simulink model "dspace"  (R2021b)
settings: Solver=FixedStepDiscrete  StartTime=0.0  StopTime=Inf  FixedStep=1e-3  RelTol=1e-3
PostLoadFcn:
  | , if any(exist('dsrtsu_mdlpostloadfcn', 'file') ~= 0), dsrtsu_mdlpostloadfcn('Execute', bdroot); end,
undefined symbols (not defined in the file): ami, amk1_setpoints_1, amk2_setpoints_1, amk3_setpoints_1, amk4_setpoints_1, as, digital, ebs, indicator, mcu_set_dbu_indicator_points, mcu_set_ecu_indicator_points, res_ntm_node_control
libraries: rtican x63, rti1401lib_dio_type3 x4, simulink x4, simulink_extras x1
(part 7 of 16)

== system dspace/CAN RX/amk4_actual_values_1 ==
  amk4_actual_values_11 : rtican/RTICAN Receive (RX)   Reserved1=[]  Reserved2=[]  Reserved3=[]  Reserved4=[]  SfcnMessage=[]  Msg_Struct=[]  BoardTypeNo=[]  BoardNo=[]  ChannelNo=[]  Parameters=[]  DialogFcn=[]  UnitName=[]  Revision=[]  UnitValues=[]  DSProperties=struct('RTI',struct('Version',uint32(5),'BlockType',struct('isSLSource',uint8(1),'isSLSink',uint8(1),'isHWSource',uint8(0),'isHWSink',uint8(0),'isSetup',uint8(0),'isInline',uint8(1),'isNonInline',uint8(0),'isInterrupt',uint8(0),'isChannelwise',uint8(0)),'IOBoardType','RTICAN','UnitType','MESSAGE','Identifier','RX','DialogType','MSVC','BlockSet','RTICAN','SlaveProcessor','CAN'))  RTIBlockInterface=struct('OutputPortsWidth',int32([1 1 1 1 1 1 1 1 1 1 1 1 1 1]),'OutputPortsActive',ones(1,14),'OutputPortsName',{{'amk4_system_ready','amk4_error','amk4_warning','amk4_status_quit_dc_on','amk4_status_dc_on','amk4_status_quit_inverter_on','amk4_status_inverter_on','amk4_status_derating','amk4_actual_velocity','amk4_torque_current','amk4_magnetizing_current',['RX status'],['RX time'],['RX delta time']}},'OutputPortsDataType',{{'SS_DOUBLE','SS_DOUBLE','SS_DOUBLE','SS_DOUBLE','SS_DOUBLE','SS_DOUBLE','SS_DOUBLE','SS_DOUBLE','SS_DOUBLE','SS_DOUBLE','SS_DOUBLE','SS_DOUBLE','SS_DOUBLE','SS_DOUBLE'}},'OutputPortsLabel',{{'amk4_system_ready','amk4_error','amk4_warning','amk4_status_quit_dc_on','amk4_status_dc_on','amk4_status_quit_inverter_on','amk4_status_inverter_on','amk4_status_derating','amk4_actual_velocity','amk4_torque_current','amk4_magnetizing_current','','',''}},'OutputPortsLabelMode','ON','InputPortsWidth',int32(0),'InputPortsActive',0,'DialogFcn','rtican_message_interface_gui','BlockDisplay',{{'','center'}},'IconTransparency','on','ParameterTunableNames',{{}},'InitLevel',3,'BlockName',struct('Token',{{'amk4_actual_values_1'}}),'SampleTime',{{-1}},'TriggerPort',{{'none'}},'EnablePort',{{'none'}})  RTIBlockParameters=struct('BoardTypeNo',{{1,'OFF',[]}},'BoardNo',{{1,'ON',[1 16]}},'ChannelNo',{{1,'ON',[1 2]}},'Parameters',{{struct('DataFileSupport',struct('DataFileSelectedMaster',1,'DataFileSelectedLocal',1,'DataFileName','c:\users\oscar\documents\github\sw_infrastructure\kthfspe_python\databases\can2.dbc|','DataFileDate',{{{['10-Jul-2022 04:24:51']}}},'SelectedFile','c:\users\oscar\documents\github\sw_infrastructure\kthfspe_python\databases\can2.dbc'),'Options',struct('StatusSelected',1,'TimeSelected',1,'DeltaTimeSelected',1,'BytePortSelected',0,'MessageLengthSelected',0,'TriggerPort',struct('Selected',0,'TriggerType',0),'UserCoding',struct('Selected',0,'InterfaceFile','UserDecodingFile','FcnName','UserDecodeFcn','InportSelected',0,'InportWidth',1,'OutportSelected',0,'OutportWidth',1),'EnablePortSelected',0,'SignalOnPortnameSelected',1,'UseRXService',0),'Message',struct('MsgOnBlocknameSelected',1,'MsgName','amk4_actual_values_1','MsgIdFormat',0,'MsgId',648,'MsgLength',8,'NumSignals',11,'SampleTime',-1,'Signal',struct('SgnName',{'amk4_system_ready','amk4_error','amk4_warning','amk4_status_quit_dc_on','amk4_status_dc_on','amk4_status_quit_inverter_on','amk4_status_inverter_on','amk4_status_derating','amk4_actual_velocity','amk4_torque_current','amk4_magnetizing_current'},'SgnStartBit',{8,9,10,11,12,13,14,15,16,32,48},'SgnLength',{1,1,1,1,1,1,1,1,16,16,16},'SgnType',{0,0,0,0,0,0,0,0,0,0,0},'ModeValue',{-1,-1,-1,-1,-1,-1,-1,-1,-1,-1,-1},'DataType',{0,0,0,0,0,0,0,0,1,1,1},'ByteLayout',{0,0,0,0,0,0,0,0,0,0,0},'Factor',{1,1,1,1,1,1,1,1,1,1,1},'Offset',{0,0,0,0,0,0,0,0,0,0,0},'SgnComment',{{''},{''},{''},{''},{''},{''},{''},{''},{''},{''},{''}},'SgnUnit',{'','','','','','','','','rpm','',''},'Min',{0,0,0,0,0,0,0,0,0,0,0},'Max',{0,0,0,0,0,0,0,0,0,0,0},'SLDataType',{'SS_DOUBLE','SS_DOUBLE','SS_DOUBLE','SS_DOUBLE','SS_DOUBLE','SS_DOUBLE','SS_DOUBLE','SS_DOUBLE','SS_DOUBLE','SS_DOUBLE','SS_DOUBLE'}),'MsgIdNumFormat',0,'MsgComment',{{['Periodic 5ms.']}}),'Version',1.2,'general',struct('isFromLib',0)),'OFF',[]}},'GroupId',{{struct('Group',{{'RTICAN'}},'No',2,'Behavior',{{'NAMECHANGE'}},'BlockType',{{'SINK'}},'NameChangeFlag',0),'OFF',[]}},'SFcnRTICANMessage',{{struct('MsgType','RX','SFcnPortType','Scalar','MsgName','amk4_actual_values_1','MsgIdFormat','STD','MsgId',648,'MsgLength',8,'NumSignals',11,'SampleTime',-1,'Signal',struct('SgnName',{'amk4_system_ready','amk4_error','amk4_warning','amk4_status_quit_dc_on','amk4_status_dc_on','amk4_status_quit_inverter_on','amk4_status_inverter_on','amk4_status_derating','amk4_actual_velocity','amk4_torque_current','amk4_magnetizing_current'},'SgnStartBit',{8,9,10,11,12,13,14,15,16,32,48},'SgnLength',{1,1,1,1,1,1,1,1,16,16,16},'SgnType',{'standard','standard','standard','standard','standard','standard','standard','standard','standard','standard','standard'},'ModeValue',{-1,-1,-1,-1,-1,-1,-1,-1,-1,-1,-1},'DataType',{['unsigned int'],['unsigned int'],['unsigned int'],['unsigned int'],['unsigned int'],['unsigned int'],['unsigned int'],['unsigned int'],['signed int'],['signed int'],['signed int']},'ByteLayout',{['little endian'],['little endian'],['little endian'],['little endian'],['little endian'],['little endian'],['little endian'],['little endian'],['little endian'],['little endian'],['little endian']},'Factor',{1,1,1,1,1,1,1,1,1,1,1},'Offset',{0,0,0,0,0,0,0,0,0,0,0},'SLDataType',{'SS_DOUBLE','SS_DOUBLE','SS_DOUBLE','SS_DOUBLE','SS_DOUBLE','SS_DOUBLE','SS_DOUBLE','SS_DOUBLE','SS_DOUBLE','SS_DOUBLE','SS_DOUBLE'}),'StatusSelected','yes','TimeSelected','yes','DeltaTimeSelected','yes','BytePortSelected','no','MessageLengthSelected','no','TriggerPort',struct('Selected','no','TriggerType',0),'UserCoding',struct('Selected','no','InterfaceFile','UserDecodingFile','FcnName','UserDecodeFcn','InportSelected','no','InportWidth',1,'OutportSelected','no','OutportWidth',1),'EnablePortSelected','no','UseRXService','no','BoardType','DS1','BoardNo',1,'ControllerNo',2),'OFF',[]}},'TLCFileName',{{'rtican_rx_message','OFF',[]}})  RTISFcnParameters=struct('SFcnRTICANMessage','struct','TLCFileName','char')  RTIBlockParaDefault=struct('BoardTypeNo',4302,'BoardNo',1,'ChannelNo',1,'Parameters',struct('DataFileSupport',struct('DataFileSelectedMaster',0,'DataFileSelectedLocal',0,'DataFileName','','DataFileDate','','SelectedFile',['<no file selected>']),'Options',struct('StatusSelected',1,'TimeSelected',1,'DeltaTimeSelected',1,'BytePortSelected',0,'MessageLengthSelected',0,'TriggerPort',struct('Selected',0,'TriggerType','rising'),'UserCoding',struct('Selected',0,'InterfaceFile','UserDecodingFile','FcnName','UserDecodeFcn','InportSelected',0,'InportWidth',1,'OutportSelected',0,'OutportWidth',1),'EnablePortSelected',0,'SignalOnPortnameSelected',1,'UseRXService',0),'Message',struct('MsgOnBlocknameSelected',0,'MsgName',['RX Message'],'MsgIdFormat',0,'MsgId',100,'MsgLength',8,'NumSignals',1,'SampleTime',-1,'Signal',struct('SgnName',['RX signal'],'SgnStartBit',0,'SgnLength',8,'SgnType',0,'ModeValue',-1,'DataType',0,'SLDataType','SS_DOUBLE','ByteLayout',0,'Factor',1,'Offset',0,'Min',0,'Max',255,'SgnComment',{{}},'SgnUnit',''),'MsgIdNumFormat',0,'MsgComment',{{''}}),'Version',1.2,'general',struct('isFromLib',1)),'GroupId',struct('Group',{{'RTICAN'}},'No',1,'Behavior',{{'NAMECHANGE'}},'BlockType',{{'SINK'}},'NameChangeFlag',0),'SFcnRTICANMessage',struct('MsgType','RX','MsgName',['RX Message'],'MsgIdFormat','STD','MsgId',100,'MsgLength',8,'NumSignals',1,'SampleTime',-1,'Signal',struct('SgnName',['RX signal'],'SgnStartBit',0,'SgnLength',8,'SgnType','standard','ModeValue',-1,'DataType',['unsigned int'],'ByteLayout',['little endian'],'SLDataType','SS_DOUBLE','Factor',1,'Offset',0),'StatusSelected','yes','TimeSelected','yes','DeltaTimeSelected','yes','BytePortSelected','no','MessageLengthSelected','no','EnablePortSelected','no','UserCoding',struct('Selected','no','InterfaceFile','UserDecodingFile','FcnName','UserDecodeFcn','InportSelected','no','InportWidth',1,'OutportSelected','no','OutportWidth',1),'TriggerPort',struct('Selected','no','TriggerType','rising'),'UseRXService','no','BoardType','DS4302','BoardNo',1,'ControllerNo',1,'SFcnPortType','Scalar'),'TLCFileName','rtican_rx_message')
      settings: AttributesFormatString=Group Id: RTICAN2\n  SourceProductName=dSPACE RTI CAN Blockset
  clock_time : Clock
  sub_time : Sum  Inputs=+-
  amk4_system_ready_bus : Outport  PortName=signals  Element=amk4_system_ready
  amk4_error_bus : Outport  PortName=signals  Element=amk4_error
  amk4_warning_bus : Outport  PortName=signals  Element=amk4_warning
  amk4_status_quit_dc_on_bus : Outport  PortName=signals  Element=amk4_status_quit_dc_on
  amk4_status_dc_on_bus : Outport  PortName=signals  Element=amk4_status_dc_on
  amk4_status_quit_inverter_on_bus : Outport  PortName=signals  Element=amk4_status_quit_inverter_on
  amk4_status_inverter_on_bus : Outport  PortName=signals  Element=amk4_status_inverter_on
  amk4_status_derating_bus : Outport  PortName=signals  Element=amk4_status_derating
  amk4_actual_velocity_bus : Outport  PortName=signals  Element=amk4_actual_velocity
  amk4_torque_current_bus : Outport  PortName=signals  Element=amk4_torque_current
  amk4_magnetizing_current_bus : Outport  PortName=signals  Element=amk4_magnetizing_current
  status : Outport  Port=2
  time : Outport  Port=3
  delta : Outport  Port=4
  wires:
  clock_time/1 -> sub_time/1
  sub_time/1 -> time/1
  amk4_actual_values_11/12 -> status/1
  amk4_actual_values_11/13 -> sub_time/2
  amk4_actual_values_11/14 -> delta/1
  amk4_actual_values_11/1 -> amk4_system_ready_bus/1  "amk4_system_ready"
  amk4_actual_values_11/2 -> amk4_error_bus/1  "amk4_error"
  amk4_actual_values_11/3 -> amk4_warning_bus/1  "amk4_warning"
  amk4_actual_values_11/4 -> amk4_status_quit_dc_on_bus/1  "amk4_status_quit_dc_on"
  amk4_actual_values_11/5 -> amk4_status_dc_on_bus/1  "amk4_status_dc_on"
  amk4_actual_values_11/6 -> amk4_status_quit_inverter_on_bus/1  "amk4_status_quit_inverter_on"
  amk4_actual_values_11/7 -> amk4_status_inverter_on_bus/1  "amk4_status_inverter_on"
  amk4_actual_values_11/8 -> amk4_status_derating_bus/1  "amk4_status_derating"
  amk4_actual_values_11/9 -> amk4_actual_velocity_bus/1  "amk4_actual_velocity"
  amk4_actual_values_11/10 -> amk4_torque_current_bus/1  "amk4_torque_current"
  amk4_actual_values_11/11 -> amk4_magnetizing_current_bus/1  "amk4_magnetizing_current"

== system dspace/CAN RX/amk4_actual_values_2 ==
  amk4_actual_values_21 : rtican/RTICAN Receive (RX)   Reserved1=[]  Reserved2=[]  Reserved3=[]  Reserved4=[]  SfcnMessage=[]  Msg_Struct=[]  BoardTypeNo=[]  BoardNo=[]  ChannelNo=[]  Parameters=[]  DialogFcn=[]  UnitName=[]  Revision=[]  UnitValues=[]  DSProperties=struct('RTI',struct('Version',uint32(5),'BlockType',struct('isSLSource',uint8(1),'isSLSink',uint8(1),'isHWSource',uint8(0),'isHWSink',uint8(0),'isSetup',uint8(0),'isInline',uint8(1),'isNonInline',uint8(0),'isInterrupt',uint8(0),'isChannelwise',uint8(0)),'IOBoardType','RTICAN','UnitType','MESSAGE','Identifier','RX','DialogType','MSVC','BlockSet','RTICAN','SlaveProcessor','CAN'))  RTIBlockInterface=struct('OutputPortsWidth',int32([1 1 1 1 1 1 1]),'OutputPortsActive',[1 1 1 1 1 1 1],'OutputPortsName',{{'amk4_temp_motor','amk4_temp_inverter','amk4_error_info','amk4_temp_igbt',['RX status'],['RX time'],['RX delta time']}},'OutputPortsDataType',{{'SS_DOUBLE','SS_DOUBLE','SS_DOUBLE','SS_DOUBLE','SS_DOUBLE','SS_DOUBLE','SS_DOUBLE'}},'OutputPortsLabel',{{'amk4_temp_motor','amk4_temp_inverter','amk4_error_info','amk4_temp_igbt','','',''}},'OutputPortsLabelMode','ON','InputPortsWidth',int32(0),'InputPortsActive',0,'DialogFcn','rtican_message_interface_gui','BlockDisplay',{{'','center'}},'IconTransparency','on','ParameterTunableNames',{{}},'InitLevel',3,'BlockName',struct('Token',{{'amk4_actual_values_2'}}),'SampleTime',{{-1}},'TriggerPort',{{'none'}},'EnablePort',{{'none'}})  RTIBlockParameters=struct('BoardTypeNo',{{1,'OFF',[]}},'BoardNo',{{1,'ON',[1 16]}},'ChannelNo',{{1,'ON',[1 2]}},'Parameters',{{struct('DataFileSupport',struct('DataFileSelectedMaster',1,'DataFileSelectedLocal',1,'DataFileName','c:\users\oscar\documents\github\sw_infrastructure\kthfspe_python\databases\can2.dbc|','DataFileDate',{{{['10-Jul-2022 04:24:51']}}},'SelectedFile','c:\users\oscar\documents\github\sw_infrastructure\kthfspe_python\databases\can2.dbc'),'Options',struct('StatusSelected',1,'TimeSelected',1,'DeltaTimeSelected',1,'BytePortSelected',0,'MessageLengthSelected',0,'TriggerPort',struct('Selected',0,'TriggerType',0),'UserCoding',struct('Selected',0,'InterfaceFile','UserDecodingFile','FcnName','UserDecodeFcn','InportSelected',0,'InportWidth',1,'OutportSelected',0,'OutportWidth',1),'EnablePortSelected',0,'SignalOnPortnameSelected',1,'UseRXService',0),'Message',struct('MsgOnBlocknameSelected',1,'MsgName','amk4_actual_values_2','MsgIdFormat',0,'MsgId',656,'MsgLength',8,'NumSignals',4,'SampleTime',-1,'Signal',struct('SgnName',{'amk4_temp_motor','amk4_temp_inverter','amk4_error_info','amk4_temp_igbt'},'SgnStartBit',{0,16,32,48},'SgnLength',{16,16,16,16},'SgnType',{0,0,0,0},'ModeValue',{-1,-1,-1,-1},'DataType',{1,1,0,1},'ByteLayout',{0,0,0,0},'Factor',{0.1,0.1,1,0.1},'Offset',{0,0,0,0},'SgnComment',{{''},{''},{''},{''}},'SgnUnit',{'C','C','','C'},'Min',{0,0,0,0},'Max',{0,0,0,0},'SLDataType',{'SS_DOUBLE','SS_DOUBLE','SS_DOUBLE','SS_DOUBLE'}),'MsgIdNumFormat',0,'MsgComment',{{['Periodic 5ms.']}}),'Version',1.2,'general',struct('isFromLib',0)),'OFF',[]}},'GroupId',{{struct('Group',{{'RTICAN'}},'No',2,'Behavior',{{'NAMECHANGE'}},'BlockType',{{'SINK'}},'NameChangeFlag',0),'OFF',[]}},'SFcnRTICANMessage',{{struct('MsgType','RX','SFcnPortType','Scalar','MsgName','amk4_actual_values_2','MsgIdFormat','STD','MsgId',656,'MsgLength',8,'NumSignals',4,'SampleTime',-1,'Signal',struct('SgnName',{'amk4_temp_motor','amk4_temp_inverter','amk4_error_info','amk4_temp_igbt'},'SgnStartBit',{0,16,32,48},'SgnLength',{16,16,16,16},'SgnType',{'standard','standard','standard','standard'},'ModeValue',{-1,-1,-1,-1},'DataType',{['signed int'],['signed int'],['unsigned int'],['signed int']},'ByteLayout',{['little endian'],['little endian'],['little endian'],['little endian']},'Factor',{0.1,0.1,1,0.1},'Offset',{0,0,0,0},'SLDataType',{'SS_DOUBLE','SS_DOUBLE','SS_DOUBLE','SS_DOUBLE'}),'StatusSelected','yes','TimeSelected','yes','DeltaTimeSelected','yes','BytePortSelected','no','MessageLengthSelected','no','TriggerPort',struct('Selected','no','TriggerType',0),'UserCoding',struct('Selected','no','InterfaceFile','UserDecodingFile','FcnName','UserDecodeFcn','InportSelected','no','InportWidth',1,'OutportSelected','no','OutportWidth',1),'EnablePortSelected','no','UseRXService','no','BoardType','DS1','BoardNo',1,'ControllerNo',2),'OFF',[]}},'TLCFileName',{{'rtican_rx_message','OFF',[]}})  RTISFcnParameters=struct('SFcnRTICANMessage','struct','TLCFileName','char')  RTIBlockParaDefault=struct('BoardTypeNo',4302,'BoardNo',1,'ChannelNo',1,'Parameters',struct('DataFileSupport',struct('DataFileSelectedMaster',0,'DataFileSelectedLocal',0,'DataFileName','','DataFileDate','','SelectedFile',['<no file selected>']),'Options',struct('StatusSelected',1,'TimeSelected',1,'DeltaTimeSelected',1,'BytePortSelected',0,'MessageLengthSelected',0,'TriggerPort',struct('Selected',0,'TriggerType','rising'),'UserCoding',struct('Selected',0,'InterfaceFile','UserDecodingFile','FcnName','UserDecodeFcn','InportSelected',0,'InportWidth',1,'OutportSelected',0,'OutportWidth',1),'EnablePortSelected',0,'SignalOnPortnameSelected',1,'UseRXService',0),'Message',struct('MsgOnBlocknameSelected',0,'MsgName',['RX Message'],'MsgIdFormat',0,'MsgId',100,'MsgLength',8,'NumSignals',1,'SampleTime',-1,'Signal',struct('SgnName',['RX signal'],'SgnStartBit',0,'SgnLength',8,'SgnType',0,'ModeValue',-1,'DataType',0,'SLDataType','SS_DOUBLE','ByteLayout',0,'Factor',1,'Offset',0,'Min',0,'Max',255,'SgnComment',{{}},'SgnUnit',''),'MsgIdNumFormat',0,'MsgComment',{{''}}),'Version',1.2,'general',struct('isFromLib',1)),'GroupId',struct('Group',{{'RTICAN'}},'No',1,'Behavior',{{'NAMECHANGE'}},'BlockType',{{'SINK'}},'NameChangeFlag',0),'SFcnRTICANMessage',struct('MsgType','RX','MsgName',['RX Message'],'MsgIdFormat','STD','MsgId',100,'MsgLength',8,'NumSignals',1,'SampleTime',-1,'Signal',struct('SgnName',['RX signal'],'SgnStartBit',0,'SgnLength',8,'SgnType','standard','ModeValue',-1,'DataType',['unsigned int'],'ByteLayout',['little endian'],'SLDataType','SS_DOUBLE','Factor',1,'Offset',0),'StatusSelected','yes','TimeSelected','yes','DeltaTimeSelected','yes','BytePortSelected','no','MessageLengthSelected','no','EnablePortSelected','no','UserCoding',struct('Selected','no','InterfaceFile','UserDecodingFile','FcnName','UserDecodeFcn','InportSelected','no','InportWidth',1,'OutportSelected','no','OutportWidth',1),'TriggerPort',struct('Selected','no','TriggerType','rising'),'UseRXService','no','BoardType','DS4302','BoardNo',1,'ControllerNo',1,'SFcnPortType','Scalar'),'TLCFileName','rtican_rx_message')
      settings: AttributesFormatString=Group Id: RTICAN2\n  SourceProductName=dSPACE RTI CAN Blockset
  clock_time : Clock
  sub_time : Sum  Inputs=+-
  amk4_temp_motor_bus : Outport  PortName=signals  Element=amk4_temp_motor
  amk4_temp_inverter_bus : Outport  PortName=signals  Element=amk4_temp_inverter
  amk4_error_info_bus : Outport  PortName=signals  Element=amk4_error_info
  amk4_temp_igbt_bus : Outport  PortName=signals  Element=amk4_temp_igbt
  status : Outport  Port=2
  time : Outport  Port=3
  delta : Outport  Port=4
  wires:
  clock_time/1 -> sub_time/1
  sub_time/1 -> time/1
  amk4_actual_values_21/5 -> status/1
  amk4_actual_values_21/6 -> sub_time/2
  amk4_actual_values_21/7 -> delta/1
  amk4_actual_values_21/1 -> amk4_temp_motor_bus/1  "amk4_temp_motor"
  amk4_actual_values_21/2 -> amk4_temp_inverter_bus/1  "amk4_temp_inverter"
  amk4_actual_values_21/3 -> amk4_error_info_bus/1  "amk4_error_info"
  amk4_actual_values_21/4 -> amk4_temp_igbt_bus/1  "amk4_temp_igbt"

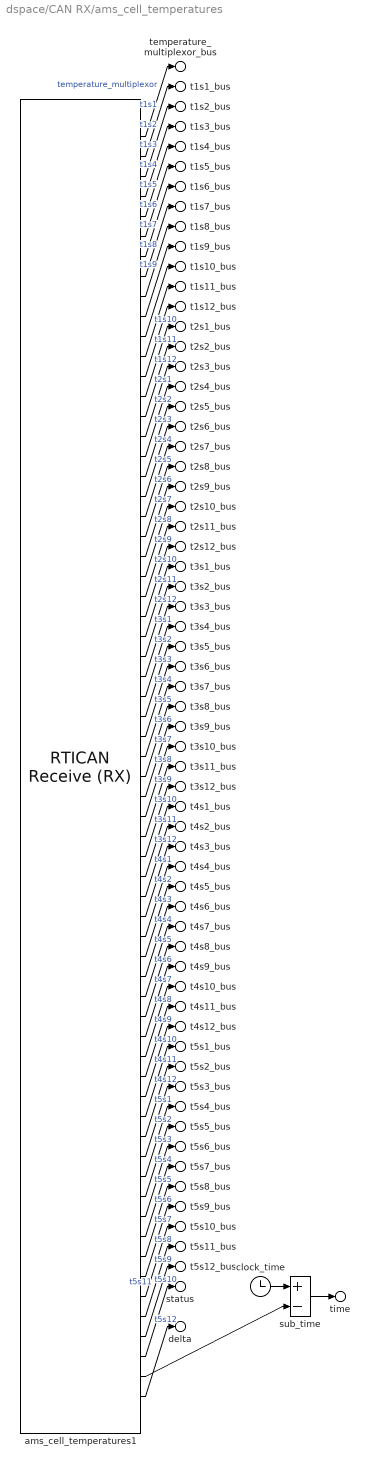
== system dspace/CAN RX/ams_cell_temperatures ==
  ams_cell_temperatures1 : rtican/RTICAN Receive (RX)   Reserved1=[]  Reserved2=[]  Reserved3=[]  Reserved4=[]  SfcnMessage=[]  Msg_Struct=[]  BoardTypeNo=[]  BoardNo=[]  ChannelNo=[]  Parameters=[]  DialogFcn=[]  UnitName=[]  Revision=[]  UnitValues=[]  DSProperties=struct('RTI',struct('Version',uint32(5),'BlockType',struct('isSLSource',uint8(1),'isSLSink',uint8(1),'isHWSource',uint8(0),'isHWSink',uint8(0),'isSetup',uint8(0),'isInline',uint8(1),'isNonInline',uint8(0),'isInterrupt',uint8(0),'isChannelwise',uint8(0)),'IOBoardType','RTICAN','UnitType','MESSAGE','Identifier','RX','DialogType','MSVC','BlockSet','RTICAN','SlaveProcessor','CAN'))  RTIBlockInterface=struct('OutputPortsWidth',int32([1 1 1 1 1 1 1 1 1 1 1 1 1 1 1 1 1 1 1 1 1 1 1 1 1 1 1 1 1 1 1 1 1 1 1 1 1 1 1 1 1 1 1 1 1 1 1 1 1 1 1 1 1 1 1 1 1 1 1 1 1 1 1 1]),'OutputPortsActive',ones(1,64),'OutputPortsName',{{'temperature_multiplexor','t1s1','t1s2','t1s3','t1s4','t1s5','t1s6','t1s7','t1s8','t1s9','t1s10','t1s11','t1s12','t2s1','t2s2','t2s3','t2s4','t2s5','t2s6','t2s7','t2s8','t2s9','t2s10','t2s11','t2s12','t3s1','t3s2','t3s3','t3s4','t3s5','t3s6','t3s7','t3s8','t3s9','t3s10','t3s11','t3s12','t4s1','t4s2','t4s3','t4s4','t4s5','t4s6','t4s7','t4s8','t4s9','t4s10','t4s11','t4s12','t5s1','t5s2','t5s3','t5s4','t5s5','t5s6','t5s7','t5s8','t5s9','t5s10','t5s11','t5s12',['RX status'],['RX time'],['RX delta time']}},'OutputPortsDataType',{{'SS_DOUBLE','SS_DOUBLE','SS_DOUBLE','SS_DOUBLE','SS_DOUBLE','SS_DOUBLE','SS_DOUBLE','SS_DOUBLE','SS_DOUBLE','SS_DOUBLE','SS_DOUBLE','SS_DOUBLE','SS_DOUBLE','SS_DOUBLE','SS_DOUBLE','SS_DOUBLE','SS_DOUBLE','SS_DOUBLE','SS_DOUBLE','SS_DOUBLE','SS_DOUBLE','SS_DOUBLE','SS_DOUBLE','SS_DOUBLE','SS_DOUBLE','SS_DOUBLE','SS_DOUBLE','SS_DOUBLE','SS_DOUBLE','SS_DOUBLE','SS_DOUBLE','SS_DOUBLE','SS_DOUBLE','SS_DOUBLE','SS_DOUBLE','SS_DOUBLE','SS_DOUBLE','SS_DOUBLE','SS_DOUBLE','SS_DOUBLE','SS_DOUBLE','SS_DOUBLE','SS_DOUBLE','SS_DOUBLE','SS_DOUBLE','SS_DOUBLE','SS_DOUBLE','SS_DOUBLE','SS_DOUBLE','SS_DOUBLE','SS_DOUBLE','SS_DOUBLE','SS_DOUBLE','SS_DOUBLE','SS_DOUBLE','SS_DOUBLE','SS_DOUBLE','SS_DOUBLE','SS_DOUBLE','SS_DOUBLE','SS_DOUBLE','SS_DOUBLE','SS_DOUBLE','SS_DOUBLE'}},'OutputPortsLabel',{{'temperature_multiplexor','t1s1','t1s2','t1s3','t1s4','t1s5','t1s6','t1s7','t1s8','t1s9','t1s10','t1s11','t1s12','t2s1','t2s2','t2s3','t2s4','t2s5','t2s6','t2s7','t2s8','t2s9','t2s10','t2s11','t2s12','t3s1','t3s2','t3s3','t3s4','t3s5','t3s6','t3s7','t3s8','t3s9','t3s10','t3s11','t3s12','t4s1','t4s2','t4s3','t4s4','t4s5','t4s6','t4s7','t4s8','t4s9','t4s10','t4s11','t4s12','t5s1','t5s2','t5s3','t5s4','t5s5','t5s6','t5s7','t5s8','t5s9','t5s10','t5s11','t5s12','','',''}},'OutputPortsLabelMode','ON','InputPortsWidth',int32(0),'InputPortsActive',0,'DialogFcn','rtican_message_interface_gui','BlockDisplay',{{'','center'}},'IconTransparency','on','ParameterTunableNames',{{}},'InitLevel',3,'BlockName',struct('Token',{{'ams_cell_temperatures'}}),'SampleTime',{{-1}},'TriggerPort',{{'none'}},'EnablePort',{{'none'}})  RTIBlockParameters=struct('BoardTypeNo',{{1,'OFF',[]}},'BoardNo',{{1,'ON',[1 16]}},'ChannelNo',{{2,'ON',[1 2]}},'Parameters',{{struct('DataFileSupport',struct('DataFileSelectedMaster',1,'DataFileSelectedLocal',1,'DataFileName','c:\users\oscar\documents\github\sw_infrastructure\kthfspe_python\databases\can1.dbc|','DataFileDate',{{{['10-Jul-2022 16:14:04']}}},'SelectedFile','c:\users\oscar\documents\github\sw_infrastructure\kthfspe_python\databases\can1.dbc'),'Options',struct('StatusSelected',1,'TimeSelected',1,'DeltaTimeSelected',1,'BytePortSelected',0,'MessageLengthSelected',0,'TriggerPort',struct('Selected',0,'TriggerType',0),'UserCoding',struct('Selected',0,'InterfaceFile','UserDecodingFile','FcnName','UserDecodeFcn','InportSelected',0,'InportWidth',1,'OutportSelected',0,'OutportWidth',1),'EnablePortSelected',0,'SignalOnPortnameSelected',1,'UseRXService',0),'Message',struct('MsgOnBlocknameSelected',1,'MsgName','ams_cell_temperatures','MsgIdFormat',0,'MsgId',34,'MsgLength',8,'NumSignals',61,'SampleTime',-1,'Signal',struct('SgnName',{'temperature_multiplexor','t1s1','t1s2','t1s3','t1s4','t1s5','t1s6','t1s7','t1s8','t1s9','t1s10','t1s11','t1s12','t2s1','t2s2','t2s3','t2s4','t2s5','t2s6','t2s7','t2s8','t2s9','t2s10','t2s11','t2s12','t3s1','t3s2','t3s3','t3s4','t3s5','t3s6','t3s7','t3s8','t3s9','t3s10','t3s11','t3s12','t4s1','t4s2','t4s3','t4s4','t4s5','t4s6','t4s7','t4s8','t4s9','t4s10','t4s11','t4s12','t5s1','t5s2','t5s3','t5s4','t5s5','t5s6','t5s7','t5s8','t5s9','t5s10','t5s11','t5s12'},'SgnStartBit',{0,4,4,4,4,4,4,4,4,4,4,4,4,16,16,16,16,16,16,16,16,16,16,16,16,28,28,28,28,28,28,28,28,28,28,28,28,40,40,40,40,40,40,40,40,40,40,40,40,52,52,52,52,52,52,52,52,52,52,52,52},'SgnLength',{4,12,12,12,12,12,12,12,12,12,12,12,12,12,12,12,12,12,12,12,12,12,12,12,12,12,12,12,12,12,12,12,12,12,12,12,12,12,12,12,12,12,12,12,12,12,12,12,12,12,12,12,12,12,12,12,12,12,12,12,12},'SgnType',{1,2,2,2,2,2,2,2,2,2,2,2,2,2,2,2,2,2,2,2,2,2,2,2,2,2,2,2,2,2,2,2,2,2,2,2,2,2,2,2,2,2,2,2,2,2,2,2,2,2,2,2,2,2,2,2,2,2,2,2,2},'ModeValue',{-1,0,1,2,3,4,5,6,7,8,9,10,11,0,1,2,3,4,5,6,7,8,9,10,11,0,1,2,3,4,5,6,7,8,9,10,11,0,1,2,3,4,5,6,7,8,9,10,11,0,1,2,3,4,5,6,7,8,9,10,11},'DataType',{0,1,1,1,1,1,1,1,1,1,1,1,1,1,1,1,1,1,1,1,1,1,1,1,1,1,1,1,1,1,1,1,1,1,1,1,1,1,1,1,1,1,1,1,1,1,1,1,1,1,1,1,1,1,1,1,1,1,1,1,1},'ByteLayout',{0,0,0,0,0,0,0,0,0,0,0,0,0,0,0,0,0,0,0,0,0,0,0,0,0,0,0,0,0,0,0,0,0,0,0,0,0,0,0,0,0,0,0,0,0,0,0,0,0,0,0,0,0,0,0,0,0,0,0,0,0},'Factor',{1,0.04884,0.04884,0.04884,0.04884,0.04884,0.04884,0.04884,0.04884,0.04884,0.04884,0.04884,0.04884,0.04884,0.04884,0.04884,0.04884,0.04884,0.04884,0.04884,0.04884,0.04884,0.04884,0.04884,0.04884,0.04884,0.04884,0.04884,0.04884,0.04884,0.04884,0.04884,0.04884,0.04884,0.04884,0.04884,0.04884,0.04884,0.04884,0.04884,0.04884,0.04884,0.04884,0.04884,0.04884,0.04884,0.04884,0.04884,0.04884,0.04884,0.04884,0.04884,0.04884,0.04884,0.04884,0.04884,0.04884,0.04884,0.04884,0.04884,0.04884},'Offset',{0,-10,-10,-10,-10,-10,-10,-10,-10,-10,-10,-10,-10,-10,-10,-10,-10,-10,-10,-10,-10,-10,-10,-10,-10,-10,-10,-10,-10,-10,-10,-10,-10,-10,-10,-10,-10,-10,-10,-10,-10,-10,-10,-10,-10,-10,-10,-10,-10,-10,-10,-10,-10,-10,-10,-10,-10,-10,-10,-10,-10},'SgnComment',{{''},{''},{''},{''},{''},{''},{''},{''},{''},{''},{''},{''},{''},{''},{''},{''},{''},{''},{''},{''},{''},{''},{''},{''},{''},{''},{''},{''},{''},{''},{''},{''},{''},{''},{''},{''},{''},{''},{''},{''},{''},{''},{''},{''},{''},{''},{''},{''},{''},{''},{''},{''},{''},{''},{''},{''},{''},{''},{''},{''},{''}},'SgnUnit',{'','C','C','C','C','C','C','C','C','C','C','C','C','C','C','C','C','C','C','C','C','C','C','C','C','C','C','C','C','C','C','C','C','C','C','C','C','C','C','C','C','C','C','C','C','C','C','C','C','C','C','C','C','C','C','C','C','C','C','C','C'},'Min',{0,-10,-10,-10,-10,-10,-10,-10,-10,-10,-10,-10,-10,-10,-10,-10,-10,-10,-10,-10,-10,-10,-10,-10,-10,-10,-10,-10,-10,-10,-10,-10,-10,-10,-10,-10,-10,-10,-10,-10,-10,-10,-10,-10,-10,-10,-10,-10,-10,-10,-10,-10,-10,-10,-10,-10,-10,-10,-10,-10,-10},'Max',{0,190,190,190,190,190,190,190,190,190,190,190,190,190,190,190,190,190,190,190,190,190,190,190,190,190,190,190,190,190,190,190,190,190,190,190,190,190,190,190,190,190,190,190,190,190,190,190,190,190,190,190,190,190,190,190,190,190,190,190,190},'SLDataType',{'SS_DOUBLE','SS_DOUBLE','SS_DOUBLE','SS_DOUBLE','SS_DOUBLE','SS_DOUBLE','SS_DOUBLE','SS_DOUBLE','SS_DOUBLE','SS_DOUBLE','SS_DOUBLE','SS_DOUBLE','SS_DOUBLE','SS_DOUBLE','SS_DOUBLE','SS_DOUBLE','SS_DOUBLE','SS_DOUBLE','SS_DOUBLE','SS_DOUBLE','SS_DOUBLE','SS_DOUBLE','SS_DOUBLE','SS_DOUBLE','SS_DOUBLE','SS_DOUBLE','SS_DOUBLE','SS_DOUBLE','SS_DOUBLE','SS_DOUBLE','SS_DOUBLE','SS_DOUBLE','SS_DOUBLE','SS_DOUBLE','SS_DOUBLE','SS_DOUBLE','SS_DOUBLE','SS_DOUBLE','SS_DOUBLE','SS_DOUBLE','SS_DOUBLE','SS_DOUBLE','SS_DOUBLE','SS_DOUBLE','SS_DOUBLE','SS_DOUBLE','SS_DOUBLE','SS_DOUBLE','SS_DOUBLE','SS_DOUBLE','SS_DOUBLE','SS_DOUBLE','SS_DOUBLE','SS_DOUBLE','SS_DOUBLE','SS_DOUBLE','SS_DOUBLE','SS_DOUBLE','SS_DOUBLE','SS_DOUBLE','SS_DOUBLE'}),'MsgIdNumFormat',0,'MsgComment',{{''}}),'Version',1.2,'general',struct('isFromLib',0)),'OFF',[]}},'GroupId',{{struct('Group',{{'RTICAN'}},'No',1,'Behavior',{{'NAMECHANGE'}},'BlockType',{{'SINK'}},'NameChangeFlag',0),'OFF',[]}},'SFcnRTICANMessage',{{struct('MsgType','RX','SFcnPortType','Scalar','MsgName','ams_cell_temperatures','MsgIdFormat','STD','MsgId',34,'MsgLength',8,'NumSignals',61,'SampleTime',-1,'Signal',struct('SgnName',{'temperature_multiplexor','t1s1','t1s2','t1s3','t1s4','t1s5','t1s6','t1s7','t1s8','t1s9','t1s10','t1s11','t1s12','t2s1','t2s2','t2s3','t2s4','t2s5','t2s6','t2s7','t2s8','t2s9','t2s10','t2s11','t2s12','t3s1','t3s2','t3s3','t3s4','t3s5','t3s6','t3s7','t3s8','t3s9','t3s10','t3s11','t3s12','t4s1','t4s2','t4s3','t4s4','t4s5','t4s6','t4s7','t4s8','t4s9','t4s10','t4s11','t4s12','t5s1','t5s2','t5s3','t5s4','t5s5','t5s6','t5s7','t5s8','t5s9','t5s10','t5s11','t5s12'},'SgnStartBit',{0,4,4,4,4,4,4,4,4,4,4,4,4,16,16,16,16,16,16,16,16,16,16,16,16,28,28,28,28,28,28,28,28,28,28,28,28,40,40,40,40,40,40,40,40,40,40,40,40,52,52,52,52,52,52,52,52,52,52,52,52},'SgnLength',{4,12,12,12,12,12,12,12,12,12,12,12,12,12,12,12,12,12,12,12,12,12,12,12,12,12,12,12,12,12,12,12,12,12,12,12,12,12,12,12,12,12,12,12,12,12,12,12,12,12,12,12,12,12,12,12,12,12,12,12,12},'SgnType',{'mode','mode-dependent','mode-dependent','mode-dependent','mode-dependent','mode-dependent','mode-dependent','mode-dependent','mode-dependent','mode-dependent','mode-dependent','mode-dependent','mode-dependent','mode-dependent','mode-dependent','mode-dependent','mode-dependent','mode-dependent','mode-dependent','mode-dependent','mode-dependent','mode-dependent','mode-dependent','mode-dependent','mode-dependent','mode-dependent','mode-dependent','mode-dependent','mode-dependent','mode-dependent','mode-dependent','mode-dependent','mode-dependent','mode-dependent','mode-dependent','mode-dependent','mode-dependent','mode-dependent','mode-dependent','mode-dependent','mode-dependent','mode-dependent','mode-dependent','mode-dependent','mode-dependent','mode-dependent','mode-dependent','mode-dependent','mode-dependent','mode-dependent','mode-dependent','mode-dependent','mode-dependent','mode-dependent','mode-dependent','mode-dependent','mode-dependent','mode-dependent','mode-dependent','mode-dependent','mode-dependent'},'ModeValue',{-1,0,1,2,3,4,5,6,7,8,9,10,11,0,1,2,3,4,5,6,7,8,9,10,11,0,1,2,3,4,5,6,7,8,9,10,11,0,1,2,3,4,5,6,7,8,9,10,11,0,1,2,3,4,5,6,7,8,9,10,11},'DataType',{['unsigned int'],['signed int'],['signed int'],['signed int'],['signed int'],['signed int'],['signed int'],['signed int'],['signed int'],['signed int'],['signed int'],['signed int'],['signed int'],['signed int'],['signed int'],['signed int'],['signed int'],['signed int'],['signed int'],['signed int'],['signed int'],['signed int'],['signed int'],['signed int'],['signed int'],['signed int'],['signed int'],['signed int'],['signed int'],['signed int'],['signed int'],['signed int'],['signed int'],['signed int'],['signed int'],['signed int'],['signed int'],['signed int'],['signed int'],['signed int'],['signed int'],['signed int'],['signed int'],['signed int'],['signed int'],['signed int'],['signed int'],['signed int'],['signed int'],['signed int'],['signed int'],['signed int'],['signed int'],['signed int'],['signed int'],['signed int'],['signed int'],['signed int'],['signed int'],['signed int'],['signed int']},'ByteLayout',{['little endian'],['little endian'],['little endian'],['little endian'],['little endian'],['little endian'],['little endian'],['little endian'],['little endian'],['little endian'],['little endian'],['little endian'],['little endian'],['little endian'],['little endian'],['little endian'],['little endian'],['little endian'],['little endian'],['little endian'],['little endian'],['little endian'],['little endian'],['little endian'],['little endian'],['little endian'],['little endian'],['little endian'],['little endian'],['little endian'],['little endian'],['little endian'],['little endian'],['little endian'],['little endian'],['little endian'],['little endian'],['little endian'],['little endian'],['little endian'],['little endian'],['little endian'],['little endian'],['little endian'],['little endian'],['little endian'],['little endian'],['little endian'],['little endian'],['little endian'],['little endian'],['little endian'],['little endian'],['little endian'],['little endian'],['little endian'],['little endian'],['little endian'],['little endian'],['little endian'],['little endian']},'Factor',{1,0.04884,0.04884,0.04884,0.04884,0.04884,0.04884,0.04884,0.04884,0.04884,0.04884,0.04884,0.04884,0.04884,0.04884,0.04884,0.04884,0.04884,0.04884,0.04884,0.04884,0.04884,0.04884,0.04884,0.04884,0.04884,0.04884,0.04884,0.04884,0.04884,0.04884,0.04884,0.04884,0.04884,0.04884,0.04884,0.04884,0.04884,0.04884,0.04884,0.04884,0.04884,0.04884,0.04884,0.04884,0.04884,0.04884,0.04884,0.04884,0.04884,0.04884,0.04884,0.04884,0.04884,0.04884,0.04884,0.04884,0.04884,0.04884,0.04884,0.04884},'Offset',{0,-10,-10,-10,-10,-10,-10,-10,-10,-10,-10,-10,-10,-10,-10,-10,-10,-10,-10,-10,-10,-10,-10,-10,-10,-10,-10,-10,-10,-10,-10,-10,-10,-10,-10,-10,-10,-10,-10,-10,-10,-10,-10,-10,-10,-10,-10,-10,-10,-10,-10,-10,-10,-10,-10,-10,-10,-10,-10,-10,-10},'SLDataType',{'SS_DOUBLE','SS_DOUBLE','SS_DOUBLE','SS_DOUBLE','SS_DOUBLE','SS_DOUBLE','SS_DOUBLE','SS_DOUBLE','SS_DOUBLE','SS_DOUBLE','SS_DOUBLE','SS_DOUBLE','SS_DOUBLE','SS_DOUBLE','SS_DOUBLE','SS_DOUBLE','SS_DOUBLE','SS_DOUBLE','SS_DOUBLE','SS_DOUBLE','SS_DOUBLE','SS_DOUBLE','SS_DOUBLE','SS_DOUBLE','SS_DOUBLE','SS_DOUBLE','SS_DOUBLE','SS_DOUBLE','SS_DOUBLE','SS_DOUBLE','SS_DOUBLE','SS_DOUBLE','SS_DOUBLE','SS_DOUBLE','SS_DOUBLE','SS_DOUBLE','SS_DOUBLE','SS_DOUBLE','SS_DOUBLE','SS_DOUBLE','SS_DOUBLE','SS_DOUBLE','SS_DOUBLE','SS_DOUBLE','SS_DOUBLE','SS_DOUBLE','SS_DOUBLE','SS_DOUBLE','SS_DOUBLE','SS_DOUBLE','SS_DOUBLE','SS_DOUBLE','SS_DOUBLE','SS_DOUBLE','SS_DOUBLE','SS_DOUBLE','SS_DOUBLE','SS_DOUBLE','SS_DOUBLE','SS_DOUBLE','SS_DOUBLE'}),'StatusSelected','yes','TimeSelected','yes','DeltaTimeSelected','yes','BytePortSelected','no','MessageLengthSelected','no','TriggerPort',struct('Selected','no','TriggerType',0),'UserCoding',struct('Selected','no','InterfaceFile','UserDecodingFile','FcnName','UserDecodeFcn','InportSelected','no','InportWidth',1,'OutportSelected','no','OutportWidth',1),'EnablePortSelected','no','UseRXService','no','BoardType','DS1','BoardNo',1,'ControllerNo',1),'OFF',[]}},'TLCFileName',{{'rtican_rx_message','OFF',[]}})  RTISFcnParameters=struct('SFcnRTICANMessage','struct','TLCFileName','char')  RTIBlockParaDefault=struct('BoardTypeNo',4302,'BoardNo',1,'ChannelNo',1,'Parameters',struct('DataFileSupport',struct('DataFileSelectedMaster',0,'DataFileSelectedLocal',0,'DataFileName','','DataFileDate','','SelectedFile',['<no file selected>']),'Options',struct('StatusSelected',1,'TimeSelected',1,'DeltaTimeSelected',1,'BytePortSelected',0,'MessageLengthSelected',0,'TriggerPort',struct('Selected',0,'TriggerType','rising'),'UserCoding',struct('Selected',0,'InterfaceFile','UserDecodingFile','FcnName','UserDecodeFcn','InportSelected',0,'InportWidth',1,'OutportSelected',0,'OutportWidth',1),'EnablePortSelected',0,'SignalOnPortnameSelected',1,'UseRXService',0),'Message',struct('MsgOnBlocknameSelected',0,'MsgName',['RX Message'],'MsgIdFormat',0,'MsgId',100,'MsgLength',8,'NumSignals',1,'SampleTime',-1,'Signal',struct('SgnName',['RX signal'],'SgnStartBit',0,'SgnLength',8,'SgnType',0,'ModeValue',-1,'DataType',0,'SLDataType','SS_DOUBLE','ByteLayout',0,'Factor',1,'Offset',0,'Min',0,'Max',255,'SgnComment',{{}},'SgnUnit',''),'MsgIdNumFormat',0,'MsgComment',{{''}}),'Version',1.2,'general',struct('isFromLib',1)),'GroupId',struct('Group',{{'RTICAN'}},'No',1,'Behavior',{{'NAMECHANGE'}},'BlockType',{{'SINK'}},'NameChangeFlag',0),'SFcnRTICANMessage',struct('MsgType','RX','MsgName',['RX Message'],'MsgIdFormat','STD','MsgId',100,'MsgLength',8,'NumSignals',1,'SampleTime',-1,'Signal',struct('SgnName',['RX signal'],'SgnStartBit',0,'SgnLength',8,'SgnType','standard','ModeValue',-1,'DataType',['unsigned int'],'ByteLayout',['little endian'],'SLDataType','SS_DOUBLE','Factor',1,'Offset',0),'StatusSelected','yes','TimeSelected','yes','DeltaTimeSelected','yes','BytePortSelected','no','MessageLengthSelected','no','EnablePortSelected','no','UserCoding',struct('Selected','no','InterfaceFile','UserDecodingFile','FcnName','UserDecodeFcn','InportSelected','no','InportWidth',1,'OutportSelected','no','OutportWidth',1),'TriggerPort',struct('Selected','no','TriggerType','rising'),'UseRXService','no','BoardType','DS4302','BoardNo',1,'ControllerNo',1,'SFcnPortType','Scalar'),'TLCFileName','rtican_rx_message')
      settings: AttributesFormatString=Group Id: RTICAN1\n  SourceProductName=dSPACE RTI CAN Blockset
  clock_time : Clock
  sub_time : Sum  Inputs=+-
  temperature_multiplexor_bus : Outport  PortName=signals  Element=temperature_multiplexor
  t1s1_bus : Outport  PortName=signals  Element=t1s1
  t1s2_bus : Outport  PortName=signals  Element=t1s2
  t1s3_bus : Outport  PortName=signals  Element=t1s3
  t1s4_bus : Outport  PortName=signals  Element=t1s4
  t1s5_bus : Outport  PortName=signals  Element=t1s5
  t1s6_bus : Outport  PortName=signals  Element=t1s6
  t1s7_bus : Outport  PortName=signals  Element=t1s7
  t1s8_bus : Outport  PortName=signals  Element=t1s8
  t1s9_bus : Outport  PortName=signals  Element=t1s9
  t1s10_bus : Outport  PortName=signals  Element=t1s10
  t1s11_bus : Outport  PortName=signals  Element=t1s11
  t1s12_bus : Outport  PortName=signals  Element=t1s12
  t2s1_bus : Outport  PortName=signals  Element=t2s1
  t2s2_bus : Outport  PortName=signals  Element=t2s2
  t2s3_bus : Outport  PortName=signals  Element=t2s3
  t2s4_bus : Outport  PortName=signals  Element=t2s4
  t2s5_bus : Outport  PortName=signals  Element=t2s5
  t2s6_bus : Outport  PortName=signals  Element=t2s6
  t2s7_bus : Outport  PortName=signals  Element=t2s7
  t2s8_bus : Outport  PortName=signals  Element=t2s8
  t2s9_bus : Outport  PortName=signals  Element=t2s9
  t2s10_bus : Outport  PortName=signals  Element=t2s10
  t2s11_bus : Outport  PortName=signals  Element=t2s11
  t2s12_bus : Outport  PortName=signals  Element=t2s12
  t3s1_bus : Outport  PortName=signals  Element=t3s1
  t3s2_bus : Outport  PortName=signals  Element=t3s2
  t3s3_bus : Outport  PortName=signals  Element=t3s3
  t3s4_bus : Outport  PortName=signals  Element=t3s4
  t3s5_bus : Outport  PortName=signals  Element=t3s5
  t3s6_bus : Outport  PortName=signals  Element=t3s6
  t3s7_bus : Outport  PortName=signals  Element=t3s7
  t3s8_bus : Outport  PortName=signals  Element=t3s8
  t3s9_bus : Outport  PortName=signals  Element=t3s9
  t3s10_bus : Outport  PortName=signals  Element=t3s10
  t3s11_bus : Outport  PortName=signals  Element=t3s11
  t3s12_bus : Outport  PortName=signals  Element=t3s12
  t4s1_bus : Outport  PortName=signals  Element=t4s1
  t4s2_bus : Outport  PortName=signals  Element=t4s2
  t4s3_bus : Outport  PortName=signals  Element=t4s3
  t4s4_bus : Outport  PortName=signals  Element=t4s4
  t4s5_bus : Outport  PortName=signals  Element=t4s5
  t4s6_bus : Outport  PortName=signals  Element=t4s6
  t4s7_bus : Outport  PortName=signals  Element=t4s7
  t4s8_bus : Outport  PortName=signals  Element=t4s8
  t4s9_bus : Outport  PortName=signals  Element=t4s9
  t4s10_bus : Outport  PortName=signals  Element=t4s10
  t4s11_bus : Outport  PortName=signals  Element=t4s11
  t4s12_bus : Outport  PortName=signals  Element=t4s12
  t5s1_bus : Outport  PortName=signals  Element=t5s1
  t5s2_bus : Outport  PortName=signals  Element=t5s2
  t5s3_bus : Outport  PortName=signals  Element=t5s3
  t5s4_bus : Outport  PortName=signals  Element=t5s4
  t5s5_bus : Outport  PortName=signals  Element=t5s5
  t5s6_bus : Outport  PortName=signals  Element=t5s6
  t5s7_bus : Outport  PortName=signals  Element=t5s7
  t5s8_bus : Outport  PortName=signals  Element=t5s8
  t5s9_bus : Outport  PortName=signals  Element=t5s9
  t5s10_bus : Outport  PortName=signals  Element=t5s10
  t5s11_bus : Outport  PortName=signals  Element=t5s11
  t5s12_bus : Outport  PortName=signals  Element=t5s12
  status : Outport  Port=2
  time : Outport  Port=3
  delta : Outport  Port=4
  wires:
  clock_time/1 -> sub_time/1
  sub_time/1 -> time/1
  ams_cell_temperatures1/62 -> status/1
  ams_cell_temperatures1/63 -> sub_time/2
  ams_cell_temperatures1/64 -> delta/1
  ams_cell_temperatures1/1 -> temperature_multiplexor_bus/1  "temperature_multiplexor"
  ams_cell_temperatures1/2 -> t1s1_bus/1  "t1s1"
  ams_cell_temperatures1/3 -> t1s2_bus/1  "t1s2"
  ams_cell_temperatures1/4 -> t1s3_bus/1  "t1s3"
  ams_cell_temperatures1/5 -> t1s4_bus/1  "t1s4"
  ams_cell_temperatures1/6 -> t1s5_bus/1  "t1s5"
  ams_cell_temperatures1/7 -> t1s6_bus/1  "t1s6"
  ams_cell_temperatures1/8 -> t1s7_bus/1  "t1s7"
  ams_cell_temperatures1/9 -> t1s8_bus/1  "t1s8"
  ams_cell_temperatures1/10 -> t1s9_bus/1  "t1s9"
  ams_cell_temperatures1/11 -> t1s10_bus/1  "t1s10"
  ams_cell_temperatures1/12 -> t1s11_bus/1  "t1s11"
  ams_cell_temperatures1/13 -> t1s12_bus/1  "t1s12"
  ams_cell_temperatures1/14 -> t2s1_bus/1  "t2s1"
  ams_cell_temperatures1/15 -> t2s2_bus/1  "t2s2"
  ams_cell_temperatures1/16 -> t2s3_bus/1  "t2s3"
  ams_cell_temperatures1/17 -> t2s4_bus/1  "t2s4"
  ams_cell_temperatures1/18 -> t2s5_bus/1  "t2s5"
  ams_cell_temperatures1/19 -> t2s6_bus/1  "t2s6"
  ams_cell_temperatures1/20 -> t2s7_bus/1  "t2s7"
  ams_cell_temperatures1/21 -> t2s8_bus/1  "t2s8"
  ams_cell_temperatures1/22 -> t2s9_bus/1  "t2s9"
  ams_cell_temperatures1/23 -> t2s10_bus/1  "t2s10"
  ams_cell_temperatures1/24 -> t2s11_bus/1  "t2s11"
  ams_cell_temperatures1/25 -> t2s12_bus/1  "t2s12"
  ams_cell_temperatures1/26 -> t3s1_bus/1  "t3s1"
  ams_cell_temperatures1/27 -> t3s2_bus/1  "t3s2"
  ams_cell_temperatures1/28 -> t3s3_bus/1  "t3s3"
  ams_cell_temperatures1/29 -> t3s4_bus/1  "t3s4"
  ams_cell_temperatures1/30 -> t3s5_bus/1  "t3s5"
  ams_cell_temperatures1/31 -> t3s6_bus/1  "t3s6"
  ams_cell_temperatures1/32 -> t3s7_bus/1  "t3s7"
  ams_cell_temperatures1/33 -> t3s8_bus/1  "t3s8"
  ams_cell_temperatures1/34 -> t3s9_bus/1  "t3s9"
  ams_cell_temperatures1/35 -> t3s10_bus/1  "t3s10"
  ams_cell_temperatures1/36 -> t3s11_bus/1  "t3s11"
  ams_cell_temperatures1/37 -> t3s12_bus/1  "t3s12"
  ams_cell_temperatures1/38 -> t4s1_bus/1  "t4s1"
  ams_cell_temperatures1/39 -> t4s2_bus/1  "t4s2"
  ams_cell_temperatures1/40 -> t4s3_bus/1  "t4s3"
  ams_cell_temperatures1/41 -> t4s4_bus/1  "t4s4"
  ams_cell_temperatures1/42 -> t4s5_bus/1  "t4s5"
  ams_cell_temperatures1/43 -> t4s6_bus/1  "t4s6"
  ams_cell_temperatures1/44 -> t4s7_bus/1  "t4s7"
  ams_cell_temperatures1/45 -> t4s8_bus/1  "t4s8"
  ams_cell_temperatures1/46 -> t4s9_bus/1  "t4s9"
  ams_cell_temperatures1/47 -> t4s10_bus/1  "t4s10"
  ams_cell_temperatures1/48 -> t4s11_bus/1  "t4s11"
  ams_cell_temperatures1/49 -> t4s12_bus/1  "t4s12"
  ams_cell_temperatures1/50 -> t5s1_bus/1  "t5s1"
  ams_cell_temperatures1/51 -> t5s2_bus/1  "t5s2"
  ams_cell_temperatures1/52 -> t5s3_bus/1  "t5s3"
  ams_cell_temperatures1/53 -> t5s4_bus/1  "t5s4"
  ams_cell_temperatures1/54 -> t5s5_bus/1  "t5s5"
  ams_cell_temperatures1/55 -> t5s6_bus/1  "t5s6"
  ams_cell_temperatures1/56 -> t5s7_bus/1  "t5s7"
  ams_cell_temperatures1/57 -> t5s8_bus/1  "t5s8"
  ams_cell_temperatures1/58 -> t5s9_bus/1  "t5s9"
  ams_cell_temperatures1/59 -> t5s10_bus/1  "t5s10"
  ams_cell_temperatures1/60 -> t5s11_bus/1  "t5s11"
  ams_cell_temperatures1/61 -> t5s12_bus/1  "t5s12"
